simulink model "Blocos"  (R2020a)
settings: Solver=VariableStepAuto  StartTime=0.0  StopTime=10.0  RelTol=1e-3
values from neighbouring files (symbols this model uses):
  c1 = (0.1)/9    (= 0.0111111111111)    [Q1-2-3.m]    (also in Q4.m)
  c2 = 1/9    (= 0.111111111111)    [Q1-2-3.m]    (also in Q4.m)
  l1 = nthroot(9,3)    [Q1-2-3.m]    (also in Q4.m)
  r1 = sqrt(9/10)    [Q1-2-3.m]    (also in Q4.m)
  r2 = 9    [Q1-2-3.m]    (also in Q4.m)
settings Model: Creator=riant  LastModifiedBy=riant

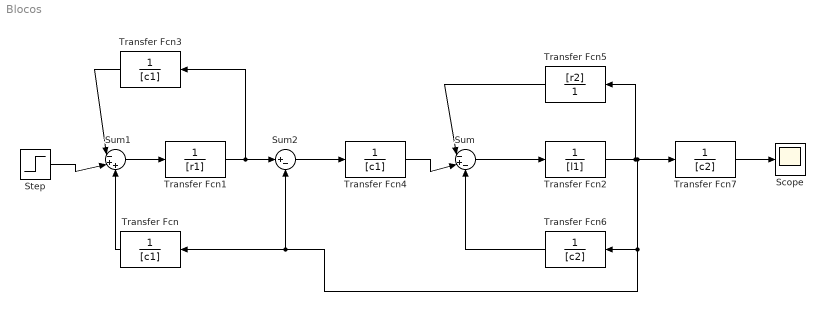
== system Blocos ==
  Scope : Scope
  Step : Step  SampleTime=0
  Sum : Sum  Inputs=|-+-
  Sum1 : Sum  Inputs=|-++
  Sum2 : Sum  Inputs=|+-
  Transfer Fcn : TransferFcn  Denominator=[c1]
  Transfer Fcn1 : TransferFcn  Denominator=[r1]
  Transfer Fcn2 : TransferFcn  Denominator=[l1]
  Transfer Fcn3 : TransferFcn  Denominator=[c1]
  Transfer Fcn4 : TransferFcn  Denominator=[c1]
  Transfer Fcn5 : TransferFcn  Numerator=[r2]  Denominator=[1]
  Transfer Fcn6 : TransferFcn  Denominator=[c2]
  Transfer Fcn7 : TransferFcn  Denominator=[c2]
  wires:
  Sum1/1 -> Transfer Fcn1/1
  Step/1 -> Sum1/2
  Transfer Fcn/1 -> Sum1/3
  Transfer Fcn3/1 -> Sum1/1
  Transfer Fcn1/1 -> Transfer Fcn3/1, Sum2/1
  Sum2/1 -> Transfer Fcn4/1
  Transfer Fcn4/1 -> Sum/2
  Sum/1 -> Transfer Fcn2/1
  Transfer Fcn6/1 -> Sum/3
  Transfer Fcn2/1 -> Transfer Fcn5/1, Transfer Fcn/1, Sum2/2, Transfer Fcn6/1, Transfer Fcn7/1
  Transfer Fcn5/1 -> Sum/1
  Transfer Fcn7/1 -> Scope/1
